simulink model "mavlinkdenemesimulink"  (R2020b)
settings: Solver=VariableStepAuto  StartTime=0.0  StopTime=10.0  RelTol=1e-3
libraries: px4uORBlib x1
settings Model: Creator=90546  LastModifiedBy=90546

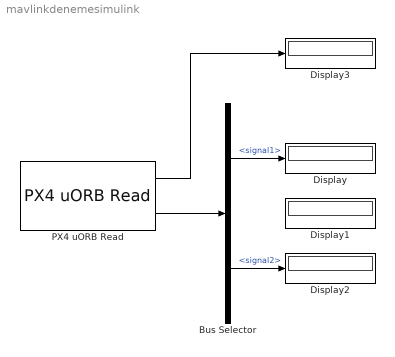
== system mavlinkdenemesimulink ==
  Bus Selector : BusSelector  OutputSignals=signal1,signal2
  Display{,1..3} (4 alike) : Display
  PX4 uORB Read : px4uORBlib/PX4 uORB Read  uORBTopic=sensor_accel  selectInstance=sensor_accel  SampleTime=0.001  BlockingMode=off  BlockTimeout=1e-3
      settings: SourceProductBaseCode=PX4AUTOPILOTS
  wires:
  PX4 uORB Read/2 -> Bus Selector/1
  PX4 uORB Read/1 -> Display3/1
  Bus Selector/1 -> Display/1  "<signal1>"
  Bus Selector/2 -> Display2/1  "<signal2>"
